simulink model "Assignment_TestGen5"  (R2017b)
settings: Solver=FixedStepDiscrete  StartTime=0.0  StopTime=10.0  RelTol=1e-3
settings Model: Creator=hbourbou  LastModifiedBy=hbourbou
settings DebuggingCC: ParameterOverflowMsg=none

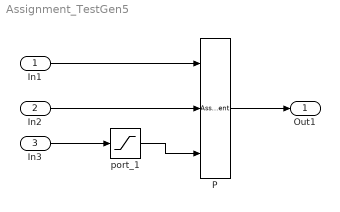
== system Assignment_TestGen5 ==
  In1 : Inport  OutDataTypeStr=single  PortDimensions=3
  In2 : Inport  Port=2  OutDataTypeStr=single  PortDimensions=2
  In3 : Inport  Port=3  OutMin=1  OutMax=2
  P : Assignment  DiagnosticForDimensions=Warning  IndexOptions=Starting index (port)  Indices=[]
  port_1 : Saturate  UpperLimit=2  LowerLimit=1
  Out1 : Outport
  wires:
  In1/1 -> P/1
  In2/1 -> P/2
  port_1/1 -> P/3
  In3/1 -> port_1/1
  P/1 -> Out1/1
